simulink model "can_bootcode_upgrade"  (Simulink 6.0)
settings: Solver=ode45  StartTime=0.0  StopTime=inf  RelTol=1e-3
libraries: canblocks x3, vector_candrivers x3, simulink x3, mpc555extras x1
settings Model: Creator=The MathWorks Inc.  LastModifiedBy=batserve  ExtModeAutoUpdateStatusClock=off  ProdHWDeviceType=Specified
settings DataIOCC: SignalLoggingName=sigsOut
settings OptimizationCC: BooleanDataType=off
settings DebuggingCC: CheckExecutionContextPreStartOutputMsg=on  CheckExecutionContextRuntimeOutputMsg=on  SolverPrmCheckMsg=none
settings HardwareCC: ProdHWDeviceType=Specified

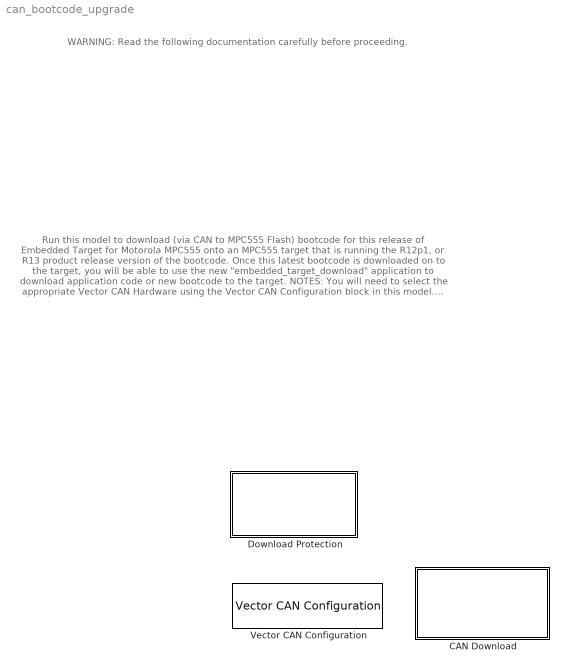
== system can_bootcode_upgrade ==
  note: Run this model to download (via CAN to MPC555 Flash) bootcode for this release
      | of Embedded Target for Motorola MPC555 onto an MPC555 target
      | that is running the R12p1, or R13 product release version of the bootcode.
      |
      | Once this latest bootcode is downloaded on to the target, you will be
      | able to use the new "embedded_target_download" application to download application
      | code or new bootcode to the target.
      |
      | NOTES:
      |
      | You will need to select the appropriate Vector CAN Hardware using the
      | Vector CAN Configuration block in this model.   Please see the documentation
      | provided on the Vector CAN blocks for more information about this.
      |
      | If this process fails, you will need to download the new bootcode via
      | the BDM port.   See the documentation for details.
      |
      | On successful completion of the download DO NOT run this model again.
      | If you do, you risk corrupting the bootcode, and you will probably have to
      | re-flash the bootcode via the BDM port.
      |
      | Please double click the "Download Protection" block to unlock the model, and then
      | run the simulation.
  note: WARNING: Read the following documentation carefully before proceeding.
  CAN Download : Subsystem  PropExecContextAcrossSSBoundary=on  mask{download_type=Flash Boot Code, download_file=0, ccp_station_id=1, ccp_cro_id=1786, ccp_dto_id=1787}
      mask prompts: download_type "Download Type"; download_file "Download Filename"; ccp_station_id "CCP Station Id"; ccp_cro_id "CCP CRO Id"; ccp_dto_id "CCP DTO Id"
      mask init:
      | % path to a bin file version of the bootcode
      | % for MPC555
      | download_file = strrep(strrep(mpc5xx_get_bootcode,'CODE_WARRIOR','DIAB'),'s19','bin');
      | if (length(download_file) > 256)
      | 	error('Download Filename longer than 256 characters.');
      | end;
      mask StyleString: popup(RAM Application Code|Flash Application Code|Flash Boot Code),edit,edit,edit,edit
      mask Display: disp('CAN Download');
  Download Protection : Subsystem  LoadFcn=|  StopFcn=|  PropExecContextAcrossSSBoundary=on
      LoadFcn=|
      | set_param(gcb,'userdata',1);           
      | set_param(gcb,'backgroundcolor','red');
      StopFcn=|
      | set_param(gcb,'userdata',1);           
      | set_param(gcb,'backgroundcolor','red');
      mask init:
      | protection=get_param(gcb,'userdata');
      | if protection==1
      | 	error('Please read the documentation, and then unlock this download model by double clicking the "Download Protection". Then try running the model again.');
      | end
      settings: OpenFcn=|
      | set_param(gcb,'userdata',0);
      | set_param(gcb,'backgroundcolor','green');
      mask Display: disp('Download Protection');
  Vector CAN Configuration : vector_candrivers/Vector CAN Configuration  tag_param=config1  channel_param=None  manual_bit_timings=off  baud_rate=500 kBaud  presc_in=1  sjw_in=1  tseg1_in=8  tseg2_in=7  sam_in=1 sample per bit

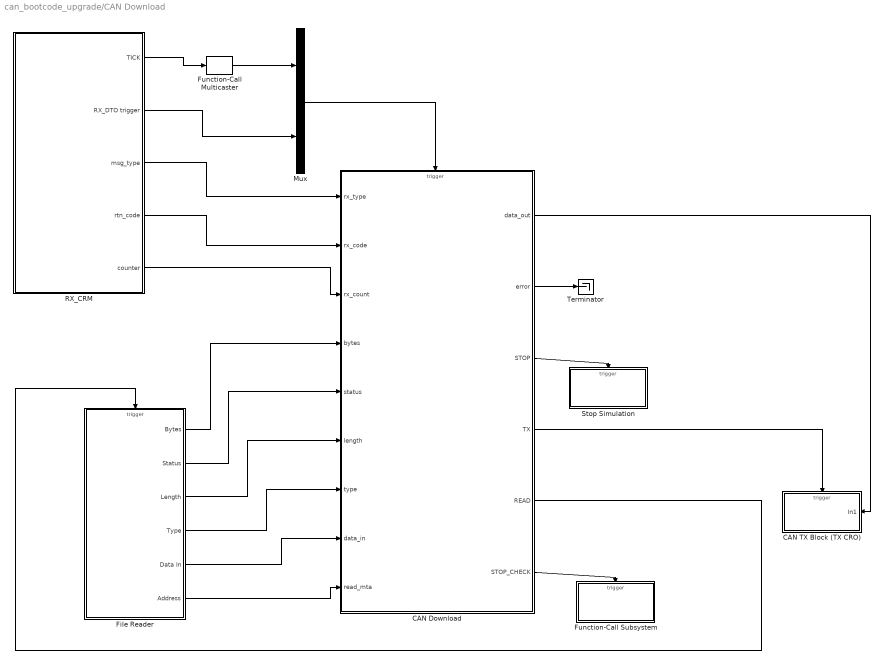
== system can_bootcode_upgrade/CAN Download ==
  CAN Download : Stateflow chart  TreatAsAtomicUnit=on  PropExecContextAcrossSSBoundary=on
  CAN TX Block (TX CRO) : Subsystem  Orientation=left  TreatAsAtomicUnit=on  PropExecContextAcrossSSBoundary=on
  File Reader : Subsystem  TreatAsAtomicUnit=on  PropExecContextAcrossSSBoundary=on
  Function-Call Multicaster : mpc555extras/Function-Call Multicaster
  Function-Call Subsystem : Subsystem  TreatAsAtomicUnit=on  PropExecContextAcrossSSBoundary=on
  Mux : Mux  Inputs=2
  RX_CRM : Subsystem  PropExecContextAcrossSSBoundary=on
  Stop Simulation : Subsystem  Orientation=left  TreatAsAtomicUnit=on  PropExecContextAcrossSSBoundary=on
  Terminator : Terminator
  wires:
  CAN Download/3(STOP) -> Stop Simulation/Trigger
  RX_CRM/5(counter) -> CAN Download/3(rx_count)
  RX_CRM/4(rtn_code) -> CAN Download/2(rx_code)
  RX_CRM/3(msg_type) -> CAN Download/1(rx_type)
  RX_CRM/2(RX_DTO trigger) -> Mux/2
  RX_CRM/1(TICK) -> Function-Call Multicaster/1
  Function-Call Multicaster/1 -> Mux/1
  Mux/1 -> CAN Download/Trigger
  CAN Download/4(TX) -> CAN TX Block (TX CRO)/Trigger
  CAN Download/1(data_out) -> CAN TX Block (TX CRO)/1(In1)
  CAN Download/5(READ) -> File Reader/Trigger
  File Reader/1(Bytes) -> CAN Download/4(bytes)
  File Reader/2(Status) -> CAN Download/5(status)
  File Reader/3(Length) -> CAN Download/6(length)
  File Reader/4(Type) -> CAN Download/7(type)
  File Reader/5(Data In) -> CAN Download/8(data_in)
  File Reader/6(Address) -> CAN Download/9(read_mta)
  CAN Download/6(STOP_CHECK) -> Function-Call Subsystem/Trigger
  CAN Download/2(error) -> Terminator/1

== system can_bootcode_upgrade/Download Protection ==

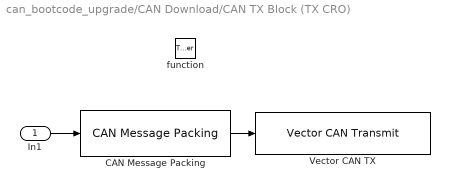
== system can_bootcode_upgrade/CAN Download/CAN TX Block (TX CRO) ==
  In1 : Inport  Port=1  LatchInput=off
  function : TriggerPort  TriggerType=function-call  StatesWhenEnabling=reset  ZeroCross=off
  CAN Message Packing : canblocks/CAN Message Packing  id=ccp_cro_id  message_type=Extended (29-bit identifier)  endian=Little Endian (Intel)
  Vector CAN TX : vector_candrivers/Vector CAN Transmit  Tag=config1  tag_param=config1  sample_time=-1
  wires:
  In1/1 -> CAN Message Packing/1
  CAN Message Packing/1 -> Vector CAN TX/1

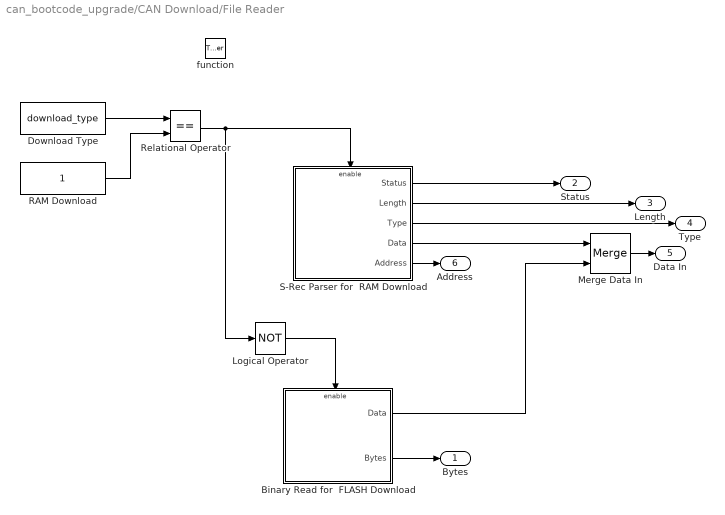
== system can_bootcode_upgrade/CAN Download/File Reader ==
  function : TriggerPort  TriggerType=function-call  StatesWhenEnabling=reset  ZeroCross=off
  Binary Read for  FLASH Download : Subsystem  TreatAsAtomicUnit=on  PropExecContextAcrossSSBoundary=on
  Download Type : Constant  Value=download_type
  Logical Operator : Logic  Operator=NOT
  Merge Data In : Merge
  RAM Download : Constant
  Relational Operator : RelationalOperator  Operator===  ZeroCross=off  InputSameDT=on
  S-Rec Parser for  RAM Download : Subsystem  TreatAsAtomicUnit=on  PropExecContextAcrossSSBoundary=on
  Bytes : Outport
  Status : Outport  Port=2
  Length : Outport  Port=3
  Type : Outport  Port=4
  Data In : Outport  Port=5
  Address : Outport  Port=6
  wires:
  S-Rec Parser for  RAM Download/4(Data) -> Merge Data In/1
  Binary Read for  FLASH Download/1(Data) -> Merge Data In/2
  Download Type/1 -> Relational Operator/1
  RAM Download/1 -> Relational Operator/2
  Relational Operator/1 -> S-Rec Parser for  RAM Download/Enable, Logical Operator/1
  Logical Operator/1 -> Binary Read for  FLASH Download/Enable
  S-Rec Parser for  RAM Download/1(Status) -> Status/1
  S-Rec Parser for  RAM Download/2(Length) -> Length/1
  S-Rec Parser for  RAM Download/3(Type) -> Type/1
  Merge Data In/1 -> Data In/1
  S-Rec Parser for  RAM Download/5(Address) -> Address/1
  Binary Read for  FLASH Download/2(Bytes) -> Bytes/1

== system can_bootcode_upgrade/CAN Download/Function-Call Subsystem ==
  function : TriggerPort  TriggerType=function-call  StatesWhenEnabling=reset  ZeroCross=off

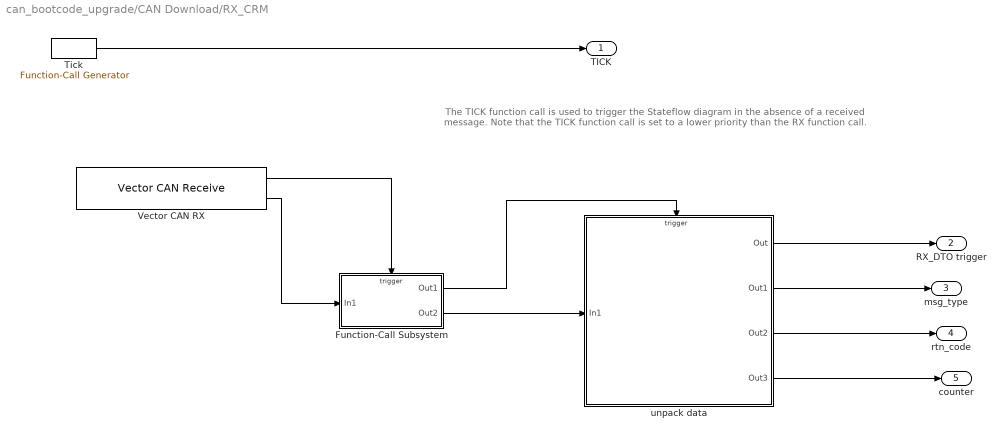
== system can_bootcode_upgrade/CAN Download/RX_CRM ==
  note: The TICK function call is used to
      | trigger the Stateflow diagram in the
      | absence of a received message. Note
      | that the TICK function call is set to a
      | lower priority than the RX function call.
  Function-Call Subsystem : Subsystem  TreatAsAtomicUnit=on  PropExecContextAcrossSSBoundary=on
  Tick : simulink/Ports & Subsystems/Function-Call Generator  Priority=3  sample_time=1  numberOfIterations=1
      settings: AttributesFormatString=Priority=%<Priority>
  Vector CAN RX : vector_candrivers/Vector CAN Receive  Tag=config1  tag_param=config1  ids=ccp_dto_id  frame_type_in=Extended (29-bit identifier)  sample_time=0.05  output_time=off  loop=off
  unpack data : Subsystem  TreatAsAtomicUnit=on  PropExecContextAcrossSSBoundary=on
  TICK : Outport
  RX_DTO trigger : Outport  Port=2
  msg_type : Outport  Port=3
  rtn_code : Outport  Port=4
  counter : Outport  Port=5
  wires:
  Tick/1 -> TICK/1
  unpack data/1(Out) -> RX_DTO trigger/1
  unpack data/2(Out1) -> msg_type/1
  unpack data/4(Out3) -> counter/1
  unpack data/3(Out2) -> rtn_code/1
  Vector CAN RX/1 -> Function-Call Subsystem/Trigger
  Vector CAN RX/2 -> Function-Call Subsystem/1(In1)
  Function-Call Subsystem/1(Out1) -> unpack data/Trigger
  Function-Call Subsystem/2(Out2) -> unpack data/1(In1)

== system can_bootcode_upgrade/CAN Download/Stop Simulation ==
  function : TriggerPort  TriggerType=function-call  StatesWhenEnabling=reset  ZeroCross=off
  Constant : Constant
  Stop Simulation : Stop
  wires:
  Constant/1 -> Stop Simulation/1

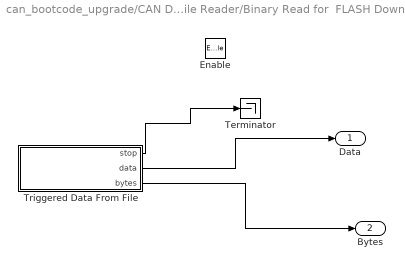
== system can_bootcode_upgrade/CAN Download/File Reader/Binary Read for  FLASH Download ==
  Enable : EnablePort  ZeroCross=off
  Terminator : Terminator
  Triggered Data From File : Subsystem  TreatAsAtomicUnit=on  PropExecContextAcrossSSBoundary=on  mask{file_name=download_file, dataType=uint8, elements=6}
      mask prompts: file_name "File Name"; elements "Number of elements per sample."
      mask help:
      | Read a binary file according to the datatype and output the data N bytes at a time. Extra zeros will be padded to the last record if the file is not divisible by N.
      |
      | This block will also stop the model when no data is left in the file so set the run time of the model to inf.
      mask init:
      | f = fopen(file_name);
      | data = fread(f,inf,['*' dataType ]);
      | fclose(f);
      | bytes = size(data,1);
      | data = [ data ; zeros(elements-rem(length(data),elements),1) ];
      | data = reshape(data,elements,[]);
      | stop = size(data,2)-1;
      mask StyleString: edit,popup(uchar|schar|int8|int16|int32|int64|uint8|uint16|uint32|single|float32|double|float64),edit
  Data : Outport
  Bytes : Outport  Port=2
  wires:
  Triggered Data From File/3(bytes) -> Bytes/1
  Triggered Data From File/2(data) -> Data/1
  Triggered Data From File/1(stop) -> Terminator/1

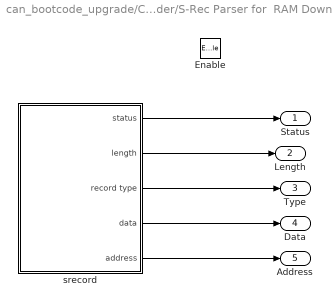
== system can_bootcode_upgrade/CAN Download/File Reader/S-Rec Parser for  RAM Download ==
  Enable : EnablePort  ZeroCross=off
  srecord : Subsystem  PropExecContextAcrossSSBoundary=on  mask{name=download_file}
      mask prompts: name "fileName"
      mask init:
      | fileName = uint8([ name zeros(1,256 - length(name))]);
  Status : Outport
  Length : Outport  Port=2
  Type : Outport  Port=3
  Data : Outport  Port=4
  Address : Outport  Port=5
  wires:
  srecord/1(status) -> Status/1
  srecord/2(length) -> Length/1
  srecord/3(record type) -> Type/1
  srecord/4(data) -> Data/1
  srecord/5(address) -> Address/1

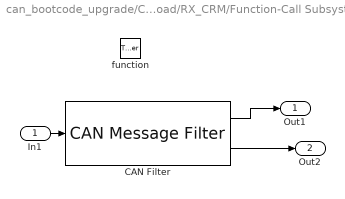
== system can_bootcode_upgrade/CAN Download/RX_CRM/Function-Call Subsystem ==
  In1 : Inport  Port=1  LatchInput=off
  function : TriggerPort  TriggerType=function-call  StatesWhenEnabling=reset  ZeroCross=off
  CAN Filter : canblocks/CAN Message Filter  id=[ccp_dto_id]
  Out1 : Outport
  Out2 : Outport  Port=2
  wires:
  In1/1 -> CAN Filter/1
  CAN Filter/1 -> Out1/1
  CAN Filter/2 -> Out2/1

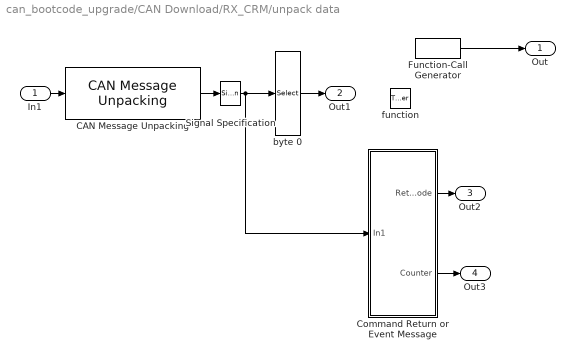
== system can_bootcode_upgrade/CAN Download/RX_CRM/unpack data ==
  In1 : Inport  Port=1  LatchInput=off
  function : TriggerPort  TriggerType=function-call  StatesWhenEnabling=reset  ZeroCross=off
  CAN Message Unpacking : canblocks/CAN Message Unpacking/CAN Message Unpacking  showData=on  showID=off  showLength=off  endian=Little Endian (Intel)
  Command Return or Event Message : Subsystem  PropExecContextAcrossSSBoundary=on
  Function-Call Generator : simulink/Ports & Subsystems/Function-Call Generator  sample_time=-1  numberOfIterations=1
  Signal Specification : SignalSpecification  Dimensions=8  DataType=uint8
  byte 0 : Selector  InputPortWidth=8
  Out : Outport
  Out1 : Outport  Port=2
  Out2 : Outport  Port=3
  Out3 : Outport  Port=4
  wires:
  Function-Call Generator/1 -> Out/1
  Command Return or Event Message/2(Counter) -> Out3/1
  Command Return or Event Message/1(Return Code) -> Out2/1
  In1/1 -> CAN Message Unpacking/1
  byte 0/1 -> Out1/1
  CAN Message Unpacking/1 -> Signal Specification/1
  Signal Specification/1 -> Command Return or Event Message/1(In1), byte 0/1

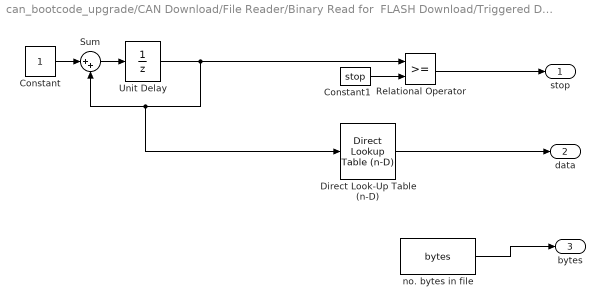
== system can_bootcode_upgrade/CAN Download/File Reader/Binary Read for  FLASH Download/Triggered Data From File ==
  Constant : Constant
  Constant1 : Constant  Value=stop
  Direct Look-Up Table (n-D) : simulink/Lookup Tables/Direct Lookup Table (n-D)  maskTabDims=2  explicitNumDims=1  outDims=Column  tabIsInput=off  mxTable=data  clipFlag=Error
  Relational Operator : RelationalOperator  ZeroCross=off  InputSameDT=on
  Sum : Sum  Inputs=|++  SaturateOnIntegerOverflow=on  InputSameDT=on
  Unit Delay : UnitDelay  SampleTime=-1
  no. bytes in file : Constant  Value=bytes
  stop : Outport
  data : Outport  Port=2
  bytes : Outport  Port=3
  wires:
  Constant/1 -> Sum/1
  Sum/1 -> Unit Delay/1
  Constant1/1 -> Relational Operator/2
  Relational Operator/1 -> stop/1
  Unit Delay/1 -> Relational Operator/1, Sum/2, Direct Look-Up Table (n-D)/1
  Direct Look-Up Table (n-D)/1 -> data/1
  no. bytes in file/1 -> bytes/1

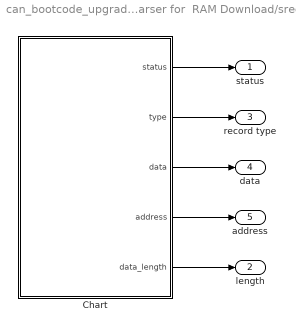
== system can_bootcode_upgrade/CAN Download/File Reader/S-Rec Parser for  RAM Download/srecord ==
  Chart : Stateflow chart  PropExecContextAcrossSSBoundary=on
  status : Outport
  length : Outport  Port=2
  record type : Outport  Port=3
  data : Outport  Port=4
  address : Outport  Port=5
  wires:
  Chart/1(status) -> status/1
  Chart/2(type) -> record type/1
  Chart/3(data) -> data/1
  Chart/4(address) -> address/1
  Chart/5(data_length) -> length/1

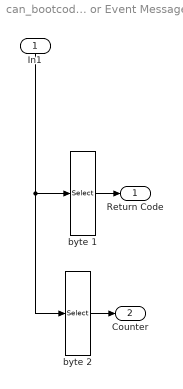
== system can_bootcode_upgrade/CAN Download/RX_CRM/unpack data/Command Return or Event Message ==
  In1 : Inport  Orientation=down  Port=1  LatchInput=off
  byte 1 : Selector  Elements=2  InputPortWidth=8
  byte 2 : Selector  Elements=3  InputPortWidth=8
  Return Code : Outport
  Counter : Outport  Port=2
  wires:
  byte 2/1 -> Counter/1
  byte 1/1 -> Return Code/1
  In1/1 -> byte 1/1, byte 2/1

== stateflow chart CAN Download/File Reader/S-Rec Parser for RAM Download/srecord/Chart ==
  settings: executeAtInitialization=1
  state File_Open
    en:status=1;
    state stop = process_data(address_size) [function]
      (junction 26) -> (junction 18) : { stop  = idx_data; }
      (junction 17) -> (junction 26) : {
          | sscanf(&buffer[idx_buffer],'%2x',&data[idx_data]);
          | idx_buffer+=2;
          | idx_data++;
          | }
      (junction 26) -> (junction 17) : [ idx_data < stop]
      (default) -> (junction 17) : {
          | idx_buffer = 2 * offset + 4;
          | idx_data = 0;
          | stop =  length  - address_size - 1;
          | }
    (junction 28) -> (junction 29)
    (junction 30) -> (junction 9) : [test != NULL ]
        | { test = sscanf(buffer,'S%1x%2x',&type,&length) ;}
    (junction 9) -> (junction 21) : [ test  == 2]
    (junction 30) -> (junction 10)
    (junction 9) -> (junction 10)
    (junction 27) -> File_Open
    (junction 11) -> (junction 28)
    (junction 21) -> (junction 20) : [ type == 1]  { sscanf(&buffer[4],'%4x',&address); offset = 2; }
    (junction 25) -> (junction 11)
    (junction 22) -> (junction 12) : [ type == 2]  { sscanf(&buffer[4],'%6x',&address); offset = 3;}
    (junction 23) -> (junction 15) : [ type == 3] { sscanf(&buffer[4],'%8x',&address); offset =4; }
    (junction 15) -> (junction 27) : { data_length = process_data(offset); }
    (junction 24) -> (junction 14) : [ type == 7]  { sscanf(&buffer[4],'%8x',&address); offset = 4;}
    (junction 12) -> (junction 15)
    (junction 25) -> (junction 16) : [ type == 8]  { sscanf(&buffer[4],'%6x',&address); offset = 3; }
    (junction 20) -> (junction 12)
    (junction 11) -> (junction 13) : [ type == 9]  { sscanf(&buffer[4],'%4x',&address); offset = 2; }
    (junction 29) -> (junction 19)
    (junction 16) -> (junction 13)
    (junction 13) -> (junction 27)
    (junction 14) -> (junction 16)
    (junction 24) -> (junction 25)
    (junction 19) -> (junction 8)
    (junction 23) -> (junction 24)
    (junction 21) -> (junction 22)
    (junction 22) -> (junction 23)
    File_Open -> (junction 8)
    (junction 8) -> (junction 30) : { test = fgets(buffer,100,file); }
  state File_Not_Open
    en:status=0
  state File_Finished
  (default) -> (junction 7) : { file = fopen(fileName,'r'); }
  (junction 7) -> File_Open
  (junction 7) -> File_Not_Open : [file ==NULL]
  (junction 10) -> File_Finished : { status = 2; }
  data: offset local double; idx_buffer temporary uint32; idx_data temporary uint32; stop function_output int32; address_size function_input double; status output uint32; type output uint32 =3; data output uint8 size=6; address output uint32; buffer local uint8 size=256; fileName local uint8 size=256; length local uint32; data_length output uint32; test local uint32

== stateflow chart CAN Download/CAN Download ==
  settings: sampleTime=1
  state success
    en:error = 0;
    en:printf('Download completed successfully.\n');
    en:STOP;
  state Programming
    state connect
      en:send_connect();
      en:connect_count++;
    state program_prepa
      en:ml('disp('' '')');
      en:ml('disp(sprintf(''Connect message acknowledged, starting download.''))');
      en:ml('disp(sprintf(''(Progress can be monitored using a CAN bus monitor)''))');
      en:ml('errorStatus = vector_can_interface(''flushtxqueues'');');
      en:send_program_prepare();
    state Flash_Download
      state Clear_Flash
        state set_mta_for_clear
          en:send_set_mta(base_offset);
        state clear_block
          en:send_clear();
        state set_mta_to_base
          en:send_set_mta(base_offset);
        clear_block -> set_mta_to_base : RX_CRM/
            | base_offset=0;
        set_mta_for_clear -> clear_block : RX_CRM
        clear_block -> set_mta_for_clear : RX_CRM[clear_iterations>1]/
            | clear_iterations--;
            | base_offset++;
      state Program_Flash
        state program6
          en:send_program6();
        state end_download
          en:send_program(0);
        state program_last_bytes
          en:send_program(last_bytes);
        (junction 121) -> program6 : [write6iterations>1]/
            | write6iterations--;
            | READ;
        program6 -> (junction 121) : RX_CRM
        (junction 121) -> program_last_bytes : [(last_bytes!=0)...
            | &...
            | (write6iterations<=1)]/
            | READ;
        program_last_bytes -> Programming.Flash_Download.Program_Flash.end_download : RX_CRM
        (junction 121) -> Programming.Flash_Download.Program_Flash.end_download : [(last_bytes==0)...
            | &...
            | (write6iterations<=1)]
      state calculate_iterations
        en:write6iterations=floor(bytes/6);
        en:last_bytes=bytes-(6*floor(bytes/6));
        en:clear_iterations = ceil(bytes/32/kb);
      set_mta_to_base -> program6 : RX_CRM/READ;
      calculate_iterations -> set_mta_for_clear
    state Ram_Download_Srec
      state end_download
        en:send_dnload(0);
      state Process_Srec_Packet
        state Execution_Start
        state Normal_Write
          state dnload
            en:send_dnload(length);
          state set_mta
            en:local_mta = read_mta + 0x800000;
            en:send_set_mta_generic(local_mta);
          state dnload6
            en:send_dnload6();
          (junction 143) -> dnload : [length>0 && length<6]
          (junction 143) -> dnload6 : [length == 6]
          dnload6 -> (junction 140) : RX_CRM
          dnload -> (junction 140) : RX_CRM
          (junction 122) -> (junction 142) : [first_time==0]
          (junction 122) -> set_mta : [first_time==1]
              | {first_time = 0;}
          set_mta -> (junction 143) : RX_CRM
          (junction 142) -> set_mta : [local_mta != (read_mta + 0x800000)]
          (junction 142) -> (junction 143) : [local_mta == (read_mta + 0x800000)]
        (junction 140) -> (junction 141) : {local_mta += length;}
        Execution_Start -> (junction 141)
        (junction 139) -> (junction 122) : [type == NORMAL_WRITE]
        (junction 139) -> Execution_Start : [type == EXECUTION_START_POINT]
      (junction 141) -> (junction 138) : {READ;}
      (junction 138) -> Programming.Ram_Download_Srec.end_download : [status == FINISHED_READING]
      (junction 138) -> (junction 139) : [status == READING]
    connect -> (junction 145) : after(1,TICK)
    (default) -> connect : {ml('disp('' '')');
        | ml('disp(sprintf(''Embedded Target for Motorola MPC555: downloading standalone real-time application.''))');
        | ml('disp('' '')');
        | ml('disp(sprintf(''To commence the CAN download, either reset the target or power it off and then back on.''))');
        | ml('disp(sprintf(''Hit Stop (Download Control Panel) or Ctrl-C (Command Window) to stop download at any time.''))');}
    connect -> program_prepa : RX_CRM
        | {connect_count=0;}
    Programming -> (junction 123) : RX_DTO
    (junction 123) -> (junction 134) : [(rx_type==CRM_type) ...
        | & ...
        | (rx_count==count)]
        | {count++;connect_count++;RX_CRM;}
    Programming.Flash_Download.Program_Flash.end_download -> (junction 135) : RX_CRM
    program_prepa -> calculate_iterations : RX_CRM
        | [(download_type == FLASH_APPLICATION_CODE)...
        | || (download_type == FLASH_BOOT_CODE)]
    program_prepa -> (junction 138) : RX_CRM
        | [download_type == RAM_APPLICATION_CODE]
        | {READ;}
    Programming.Ram_Download_Srec.end_download -> (junction 135) : RX_CRM
    (junction 145) -> connect : [connect_count==500]
        | {STOP_CHECK;
        |  connect_count=0;}
    (junction 145) -> connect
    (junction 134) -> (junction 146) : [connect_count==500]
        | {STOP_CHECK;
        | connect_count=0;}
  state failed
    en:error = 1;
    en:printf('Error during download process.\n');
    en:STOP;
  state send_set_mta_generic(address) [function]
    (default) -> (junction 144) : {data_out[0] = CCP_SET_MTA;
        |  data_out[1] = count;
        |  data_out[2] = MTA_number;
        |  data_out[3] = AddressExtension;
        |  data_out[4] = uint8(address >> 24);
        |  data_out[5] = uint8(address >> 16);
        |  data_out[6] = uint8(address >> 8);
        |  data_out[7] = uint8(address >> 0);
        |  TX;
        | }
  state send_connect() [function]
    note: Station Id (2 byte word) is processed - Intel LE format
        | Low byte first, then high byte.
    (default) -> (junction 124) : {data_out[0] = CCP_CONNECT;
        |  data_out[1] = count;
        |  data_out[2] = uint8(ccp_station_id >> 0);
        |  data_out[3] = uint8(ccp_station_id >> 8);
        |  TX;}
  state send_program_prepare() [function]
    (default) -> (junction 125) : {data_out[0] = CCP_PROGRAM_PREPARE;
        |  data_out[1] = count;}
    (junction 125) -> (junction 126) : [(download_type == RAM_APPLICATION_CODE)]
        | {data_out[2] = RAM_DOWNLOAD;}
    (junction 125) -> (junction 126) : [(download_type == FLASH_APPLICATION_CODE)...
        | || (download_type == FLASH_BOOT_CODE)]
        | {data_out[2] = FLASH_DOWNLOAD;}
    (junction 126) -> (junction 129) : {TX;}
  state send_set_mta(base_offset) [function]
    (default) -> (junction 130) : {data_out[0] = CCP_SET_MTA;
        |   data_out[1] = count;
        |   data_out[2] = MTA_number;
        |   data_out[3] = AddressExtension;}
    (junction 130) -> (junction 131) : [download_type == FLASH_APPLICATION_CODE]
        | {base = application_offset;}
    (junction 130) -> (junction 131) : [download_type == FLASH_BOOT_CODE]
        | {base = 0;}
    (junction 131) -> (junction 132) : {address = base + (base_offset * block_size);
        | data_out[4] = uint8(address >> 24);
        | data_out[5] = uint8(address >> 16);
        | data_out[6] = uint8(address >> 8);
        | data_out[7] = uint8(address >> 0);
        | TX;
        | }
  state send_clear() [function]
    (default) -> (junction 128) : {data_out[0] = CCP_CLEAR_MEMORY;
        |  data_out[1] = count;
        |  TX;}
  state send_program6() [function]
    (default) -> (junction 127) : {data_out[0] = CCP_PROGRAM_6;
        |  data_out[1] = count;
        |  data_out[2] = data_in[0];
        |  data_out[3] = data_in[1];
        |  data_out[4] = data_in[2];
        |  data_out[5] = data_in[3];
        |  data_out[6] = data_in[4];
        |  data_out[7] = data_in[5];
        |  TX;}
  state send_program(num_bytes) [function]
    (default) -> (junction 133) : {data_out[0] = CCP_PROGRAM;
        |  data_out[1] = count;
        |  data_out[2] = num_bytes;
        |  data_out[3] = data_in[0];
        |  data_out[4] = data_in[1];
        |  data_out[5] = data_in[2];
        |  data_out[6] = data_in[3];
        |  data_out[7] = data_in[4];
        |  TX;}
  state send_dnload6() [function]
    (default) -> (junction 136) : {data_out[0] = CCP_DNLOAD_6;
        |  data_out[1] = count;
        |  data_out[2] = data_in[0];
        |  data_out[3] = data_in[1];
        |  data_out[4] = data_in[2];
        |  data_out[5] = data_in[3];
        |  data_out[6] = data_in[4];
        |  data_out[7] = data_in[5];
        |  TX;}
  state send_dnload(num_bytes) [function]
    (default) -> (junction 137) : {data_out[0] = CCP_DNLOAD;
        |  data_out[1] = count;
        |  data_out[2] = num_bytes;
        |  data_out[3] = data_in[0];
        |  data_out[4] = data_in[1];
        |  data_out[5] = data_in[2];
        |  data_out[6] = data_in[3];
        |  data_out[7] = data_in[4];
        |  TX;}
  note: Functions to setup the
      | CCP packets to transmit.
  note: Failure state reached when the command return code
      | in the DTO is not 0 (== no error).   Possibilities may be
      | 0x30 == unkown command etc.   Check using a CAN
      | monitor to see what actually happened.
  note: Perform CAN download of binary data
      | to RAM or FLASH on the target.
  Programming -> failed : RX_CRM[rx_code != 0]
  (default) -> Programming
  (junction 135) -> success
  data: MTA_number constant uint8; AddressExtension constant uint8; application_offset constant uint32 =32768; base local uint32; address function_input uint32; block_size constant uint32 =32768; RAM_DOWNLOAD constant uint8; FLASH_DOWNLOAD constant uint8 =1; base_offset local uint8; base_offset function_input uint32; MTA_number constant uint8; AddressExtension constant uint8; application_offset constant uint32 =32768; base local uint32; address local uint32; block_size constant uint32 =32768; num_bytes function_input double; clear_iterations local int32; last_bytes local uint8; write6iterations local int32; kb constant int32 =1024; num_bytes function_input double; READING local uint8 =1; FINISHED_READING local double =2; first_time local boolean =1; local_mta local uint32; NORMAL_WRITE local uint8 =3; EXECUTION_START_POINT local uint8 =7; rx_type input uint8; rx_code input uint8; rx_count input uint8; CRM_type constant uint8 =255; bytes input double; data_out output uint8 size=8; error output double; RAM_APPLICATION_CODE constant uint8 =1; FLASH_APPLICATION_CODE constant uint8 =2; FLASH_BOOT_CODE constant uint8 =3; count local uint8; status input uint32; length input uint32; type input uint32; data_in input uint8 size=6; read_mta input uint32; connect_count local uint32; ccp_station_id local uint16; download_type local double
  events: TICK input FUNCTION_CALL_EVENT; RX_DTO input FUNCTION_CALL_EVENT; STOP output FUNCTION_CALL_EVENT; TX output FUNCTION_CALL_EVENT; RX_CRM local EITHER_EDGE_EVENT; READ output FUNCTION_CALL_EVENT; STOP_CHECK output FUNCTION_CALL_EVENT
